simulink model "bldc"  (R2020a)
settings: Solver=VariableStepAuto  StartTime=0.0  StopTime=10.0  RelTol=1e-3
model workspace (MAT data in the model file):
  B = Simulink.Parameter
  B.Value = 1
  B.DataType = 'auto'
  B.Dimensions = [1 1]
  J = Simulink.Parameter
  J.Value = 1
  J.DataType = 'auto'
  J.Dimensions = [1 1]
  K = Simulink.Parameter
  K.Value = 1
  K.DataType = 'auto'
  K.Dimensions = [1 1]
  L = Simulink.Parameter
  L.Value = 1
  L.DataType = 'auto'
  L.Dimensions = [1 1]
  P = Simulink.Parameter
  P.Value = 1
  P.DataType = 'auto'
  P.Dimensions = [1 1]
  R = Simulink.Parameter
  R.Value = 1
  R.DataType = 'auto'
  R.Dimensions = [1 1]
settings Model: Creator=Shivam  LastModifiedBy=Shivam

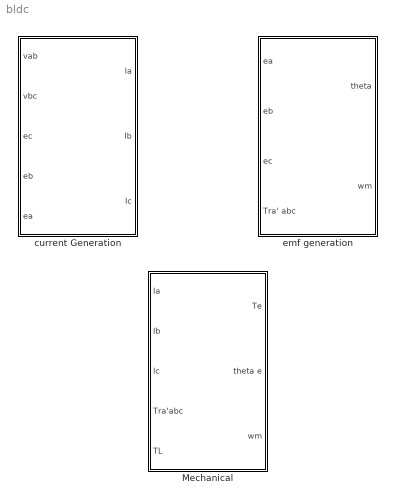
== system bldc ==
  Mechanical : Subsystem
  current Generation : Subsystem
  emf generation : Subsystem

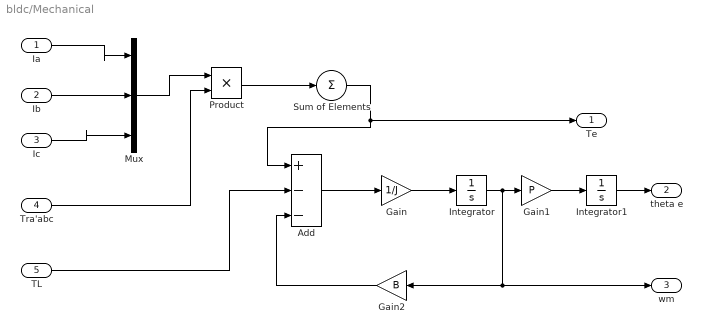
== system bldc/Mechanical ==
  Ia : Inport
  Ib : Inport  Port=2
  Ic : Inport  Port=3
  Tra'abc : Inport  Port=4
  TL : Inport  Port=5
  Add : Sum  Inputs=+--
  Gain : Gain  Gain=1/J
  Gain1 : Gain  Gain=P
  Gain2 : Gain  Gain=B
  Integrator : Integrator
  Integrator1 : Integrator
  Mux : Mux  Inputs=3
  Product : Product
  Sum of Elements : Sum  Inputs=+
  Te : Outport
  theta e : Outport  Port=2
  wm : Outport  Port=3
  wires:
  Ia/1 -> Mux/1
  Ib/1 -> Mux/2
  Ic/1 -> Mux/3
  Mux/1 -> Product/1
  Tra'abc/1 -> Product/2
  Product/1 -> Sum of Elements/1
  Sum of Elements/1 -> Add/1, Te/1
  TL/1 -> Add/2
  Add/1 -> Gain/1
  Gain/1 -> Integrator/1
  Integrator/1 -> wm/1, Gain2/1, Gain1/1
  Gain1/1 -> Integrator1/1
  Gain2/1 -> Add/3
  Integrator1/1 -> theta e/1

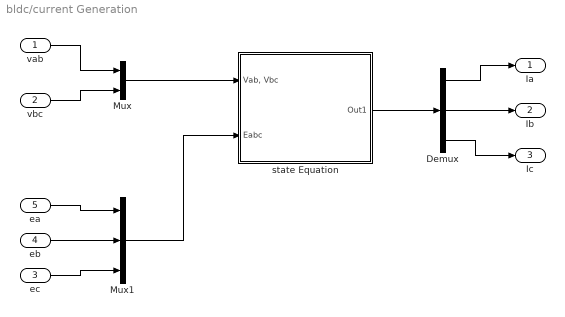
== system bldc/current Generation ==
  vab : Inport
  vbc : Inport  Port=2
  ec : Inport  Port=3
  eb : Inport  Port=4
  ea : Inport  Port=5
  Demux : Demux  Outputs=3
  Mux : Mux  Inputs=2
  Mux1 : Mux  Inputs=3
  state Equation : Subsystem
  Ia : Outport
  Ib : Outport  Port=2
  Ic : Outport  Port=3
  wires:
  vab/1 -> Mux/1
  vbc/1 -> Mux/2
  ea/1 -> Mux1/1
  eb/1 -> Mux1/2
  ec/1 -> Mux1/3
  Demux/2 -> Ib/1
  state Equation/1(Out1) -> Demux/1
  Demux/1 -> Ia/1
  Demux/3 -> Ic/1
  Mux/1 -> state Equation/1("Vab, Vbc")
  Mux1/1 -> state Equation/2(Eabc)

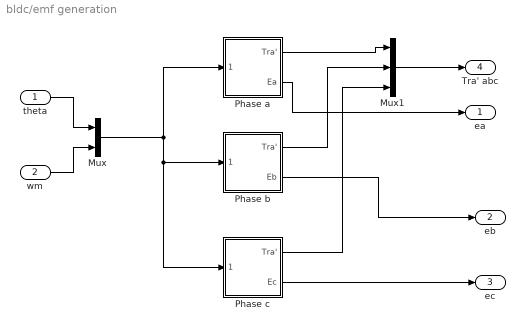
== system bldc/emf generation ==
  theta : Inport
  wm : Inport  Port=2
  Mux : Mux  Inputs=2
  Mux1 : Mux  Inputs=3
  Phase a : Subsystem
  Phase b : Subsystem
  Phase c : Subsystem
  ea : Outport
  eb : Outport  Port=2
  ec : Outport  Port=3
  Tra' abc : Outport  Port=4
  wires:
  theta/1 -> Mux/1
  wm/1 -> Mux/2
  Mux/1 -> Phase c/1(the,we), Phase b/1(the,we), Phase a/1(the,we)
  Phase c/2(Ec) -> ec/1
  Phase b/2(Eb) -> eb/1
  Phase a/2(Ea) -> ea/1
  Phase a/1(Tra') -> Mux1/1
  Phase b/1(Tra') -> Mux1/2
  Phase c/1(Tra') -> Mux1/3
  Mux1/1 -> Tra' abc/1

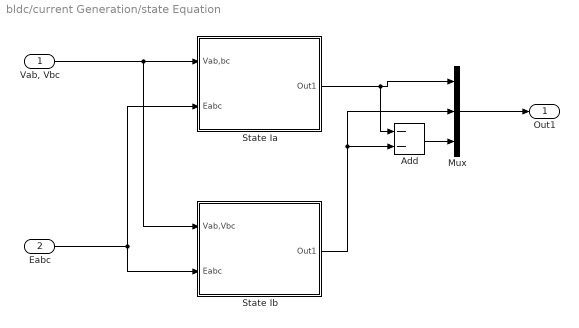
== system bldc/current Generation/state Equation ==
  "Vab, Vbc" : Inport
  Eabc : Inport  Port=2
  Add : Sum  Inputs=--
  Mux : Mux  Inputs=3
  State Ia : Subsystem
  State Ib : Subsystem
  Out1 : Outport
  wires:
  Eabc/1 -> State Ib/2(Eabc), State Ia/2(Eabc)
  "Vab, Vbc"/1 -> State Ib/1(Vab,Vbc), State Ia/1(Vab,bc)
  State Ia/1(Out1) -> Add/1, Mux/1
  State Ib/1(Out1) -> Add/2, Mux/2
  Add/1 -> Mux/3
  Mux/1 -> Out1/1

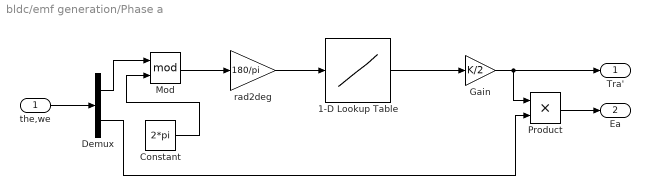
== system bldc/emf generation/Phase a ==
  the,we : Inport
  1-D Lookup Table : Lookup_n-D  NumberOfTableDimensions=1  BreakpointsForDimension1=[-5:5]  Table=tanh([-5:5])  InternalRulePriority=Speed  RndMeth=Simplest  InputSameDT=on
  Constant : Constant  Value=2*pi
  Demux : Demux  Outputs=2
  Gain : Gain  Gain=K/2
  Mod : Math  Operator=mod  SaturateOnIntegerOverflow=on
  Product : Product
  rad2deg : Gain  Gain=180/pi
  Tra' : Outport
  Ea : Outport  Port=2
  wires:
  the,we/1 -> Demux/1
  Constant/1 -> Mod/2
  Demux/1 -> Mod/1
  Mod/1 -> rad2deg/1
  rad2deg/1 -> 1-D Lookup Table/1
  Gain/1 -> Tra'/1, Product/1
  Demux/2 -> Product/2
  1-D Lookup Table/1 -> Gain/1
  Product/1 -> Ea/1

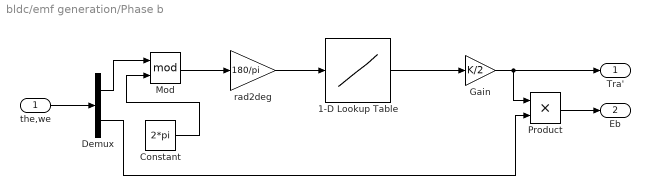
== system bldc/emf generation/Phase b ==
  the,we : Inport
  1-D Lookup Table : Lookup_n-D  NumberOfTableDimensions=1  BreakpointsForDimension1=[-5:5]  Table=tanh([-5:5])  InternalRulePriority=Speed  RndMeth=Simplest  InputSameDT=on
  Constant : Constant  Value=2*pi
  Demux : Demux  Outputs=2
  Gain : Gain  Gain=K/2
  Mod : Math  Operator=mod  SaturateOnIntegerOverflow=on
  Product : Product
  rad2deg : Gain  Gain=180/pi
  Tra' : Outport
  Eb : Outport  Port=2
  wires:
  Product/1 -> Eb/1
  Constant/1 -> Mod/2
  Gain/1 -> Tra'/1, Product/1
  Mod/1 -> rad2deg/1
  Demux/1 -> Mod/1
  1-D Lookup Table/1 -> Gain/1
  Demux/2 -> Product/2
  the,we/1 -> Demux/1
  rad2deg/1 -> 1-D Lookup Table/1

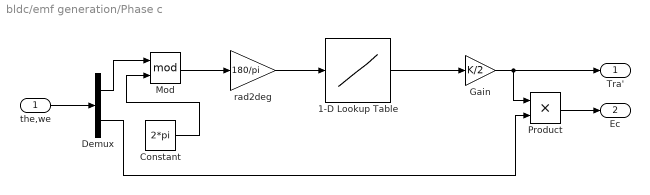
== system bldc/emf generation/Phase c ==
  the,we : Inport
  1-D Lookup Table : Lookup_n-D  NumberOfTableDimensions=1  BreakpointsForDimension1=[-5:5]  Table=tanh([-5:5])  InternalRulePriority=Speed  RndMeth=Simplest  InputSameDT=on
  Constant : Constant  Value=2*pi
  Demux : Demux  Outputs=2
  Gain : Gain  Gain=K/2
  Mod : Math  Operator=mod  SaturateOnIntegerOverflow=on
  Product : Product
  rad2deg : Gain  Gain=180/pi
  Tra' : Outport
  Ec : Outport  Port=2
  wires:
  Product/1 -> Ec/1
  Constant/1 -> Mod/2
  Gain/1 -> Tra'/1, Product/1
  Mod/1 -> rad2deg/1
  Demux/1 -> Mod/1
  1-D Lookup Table/1 -> Gain/1
  Demux/2 -> Product/2
  the,we/1 -> Demux/1
  rad2deg/1 -> 1-D Lookup Table/1

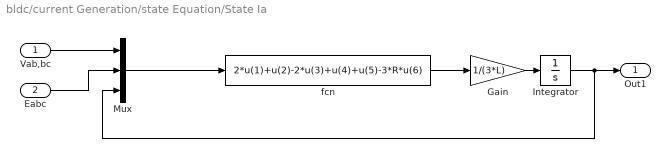
== system bldc/current Generation/state Equation/State Ia ==
  Vab,bc : Inport
  Eabc : Inport  Port=2
  Gain : Gain  Gain=1/(3*L)
  Integrator : Integrator
  Mux : Mux  Inputs=3
  fcn : Fcn  Expr=2*u(1)+u(2)-2*u(3)+u(4)+u(5)-3*R*u(6)
  Out1 : Outport
  wires:
  Vab,bc/1 -> Mux/1
  Eabc/1 -> Mux/2
  fcn/1 -> Gain/1
  Gain/1 -> Integrator/1
  Integrator/1 -> Mux/3, Out1/1
  Mux/1 -> fcn/1

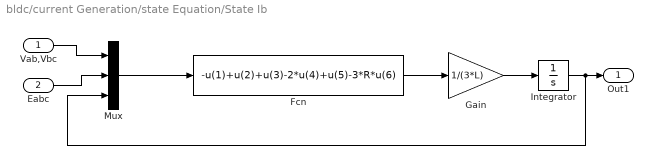
== system bldc/current Generation/state Equation/State Ib ==
  Vab,Vbc : Inport
  Eabc : Inport  Port=2
  Fcn : Fcn  Expr=-u(1)+u(2)+u(3)-2*u(4)+u(5)-3*R*u(6)
  Gain : Gain  Gain=1/(3*L)
  Integrator : Integrator
  Mux : Mux  Inputs=3
  Out1 : Outport
  wires:
  Vab,Vbc/1 -> Mux/1
  Eabc/1 -> Mux/2
  Gain/1 -> Integrator/1
  Fcn/1 -> Gain/1
  Integrator/1 -> Mux/3, Out1/1
  Mux/1 -> Fcn/1
